simulink model "ex05_target_fio2_track_object_demo"  (Simulink 7.3)
settings: Solver=FixedStepDiscrete  SolverMode=SingleTasking  StartTime=0.0  StopTime=1  RelTol=1e-3
PreLoadFcn:
  | waijung.modelPreload; % Required for working with Waijung Blockset. Do not remove.
undefined symbols (not defined in the file): A1, A2, A7, B10, B11, B12, C1, C2, C3, C4, C5, Custom, G14, H2, H3, H6, H7, Link, LQFP176, ST, STM32F417IG, system_stm32f4xx
libraries: simulink x11, stm32f4_i2c_lib x8, viptextngfix x2, stm32f4_tim_lib x2, waijung_addon_module x2, waijung_webserver x2, dspsigattribs x1, waijung_image_sensor_lib x1, stm32f4_fsmc_lib x1, stm32f4_rcc_lib x1, stm32f4_device_config_lib x1, waijung_socket_lib x1
(part 2 of 2)

== system ex05_target_fio2_track_object_demo/Image Sensor/Camera OV1/Init_/While Iterator_/Picture Size_/Subsystem/Subsystem/Img480x640 ==
  Index : Inport  OutDataType=fixdt(1, 16)  OutScaling=2^0
  Action Port : ActionPort  ActionType=default
  Register List : Subsystem  mask{register=uint8([58,61,140,64,18,50,23,24,25,26,3,12,62,112,113,114,115,162]), value=uint8([8,130,0,208,4,128,22,4,3,123,10,0,0,58,53,17,240,2])}
      mask prompts: register "Register Index"; value "Register Value"
      mask help:
      | Count:
      |  - Number of Register-Value pair.
      |  - Determine from lowest size, between Register and Value.
      | Reg:
      |  - Register index.
      | Value:
      |  - Data corresponding to specified register index.
  Count : Outport  OutDataType=fixdt(1, 16)  OutScaling=2^0
  Reg : Outport  Port=2  OutDataType=fixdt(1, 16)  OutScaling=2^0
  Value : Outport  Port=3  OutDataType=fixdt(1, 16)  OutScaling=2^0
  wires:
  Register List/3(Value) -> Value/1
  Register List/2(Reg) -> Reg/1
  Register List/1(Count) -> Count/1
  Index/1 -> Register List/1(Index)

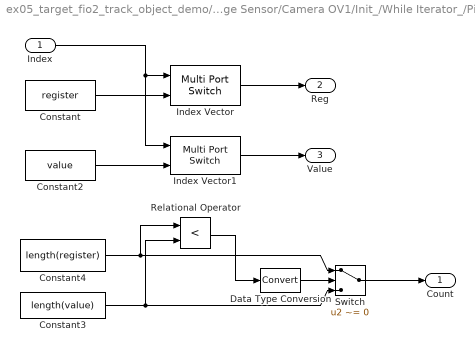
== system ex05_target_fio2_track_object_demo/Image Sensor/Camera OV1/Init_/While Iterator_/Picture Size_/Subsystem/Subsystem/Img120x160/Register List ==
  Index : Inport  OutDataType=fixdt(1, 16)  OutScaling=2^0
  Constant : Constant  Value=register  OutDataType=fixdt(1, 16)  OutScaling=2^0
  Constant2 : Constant  Value=value  OutDataType=fixdt(1, 16)  OutScaling=2^0
  Constant3 : Constant  Value=length(value)  OutDataType=fixdt(1, 16)  OutScaling=2^0
  Constant4 : Constant  Value=length(register)  OutDataType=fixdt(1, 16)  OutScaling=2^0
  Data Type Conversion : DataTypeConversion  OutDataType=fixdt(1, 16)  OutScaling=2^0
  Index Vector : MultiPortSwitch  Inputs=1  zeroidx=on  OutDataType=fixdt(1, 16)  OutScaling=2^0
  Index Vector1 : MultiPortSwitch  Inputs=1  zeroidx=on  OutDataType=fixdt(1, 16)  OutScaling=2^0
  Relational Operator : RelationalOperator  Operator=<  LogicOutDataTypeMode=boolean  LogicDataType=fixdt(0, 8)  OutDataTypeStr=boolean
  Switch : Switch  Criteria=u2 ~= 0  OutDataType=fixdt(1, 16)  OutScaling=2^0
  Count : Outport  OutDataType=fixdt(1, 16)  OutScaling=2^0
  Reg : Outport  Port=2  OutDataType=fixdt(1, 16)  OutScaling=2^0
  Value : Outport  Port=3  OutDataType=fixdt(1, 16)  OutScaling=2^0
  wires:
  Index Vector/1 -> Reg/1
  Constant/1 -> Index Vector/2
  Index/1 -> Index Vector/1, Index Vector1/1
  Constant2/1 -> Index Vector1/2
  Index Vector1/1 -> Value/1
  Constant4/1 -> Relational Operator/1, Switch/1
  Constant3/1 -> Relational Operator/2, Switch/3
  Relational Operator/1 -> Data Type Conversion/1
  Switch/1 -> Count/1
  Data Type Conversion/1 -> Switch/2

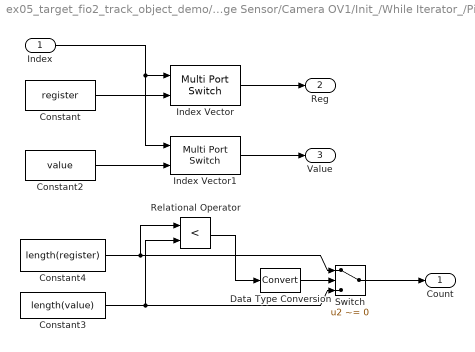
== system ex05_target_fio2_track_object_demo/Image Sensor/Camera OV1/Init_/While Iterator_/Picture Size_/Subsystem/Subsystem/Img240x320/Register List ==
  Index : Inport  OutDataType=fixdt(1, 16)  OutScaling=2^0
  Constant : Constant  Value=register  OutDataType=fixdt(1, 16)  OutScaling=2^0
  Constant2 : Constant  Value=value  OutDataType=fixdt(1, 16)  OutScaling=2^0
  Constant3 : Constant  Value=length(value)  OutDataType=fixdt(1, 16)  OutScaling=2^0
  Constant4 : Constant  Value=length(register)  OutDataType=fixdt(1, 16)  OutScaling=2^0
  Data Type Conversion : DataTypeConversion  OutDataType=fixdt(1, 16)  OutScaling=2^0
  Index Vector : MultiPortSwitch  Inputs=1  zeroidx=on  OutDataType=fixdt(1, 16)  OutScaling=2^0
  Index Vector1 : MultiPortSwitch  Inputs=1  zeroidx=on  OutDataType=fixdt(1, 16)  OutScaling=2^0
  Relational Operator : RelationalOperator  Operator=<  LogicOutDataTypeMode=boolean  LogicDataType=fixdt(0, 8)  OutDataTypeStr=boolean
  Switch : Switch  Criteria=u2 ~= 0  OutDataType=fixdt(1, 16)  OutScaling=2^0
  Count : Outport  OutDataType=fixdt(1, 16)  OutScaling=2^0
  Reg : Outport  Port=2  OutDataType=fixdt(1, 16)  OutScaling=2^0
  Value : Outport  Port=3  OutDataType=fixdt(1, 16)  OutScaling=2^0
  wires:
  Data Type Conversion/1 -> Switch/2
  Switch/1 -> Count/1
  Relational Operator/1 -> Data Type Conversion/1
  Constant3/1 -> Switch/3, Relational Operator/2
  Constant4/1 -> Switch/1, Relational Operator/1
  Index Vector1/1 -> Value/1
  Constant2/1 -> Index Vector1/2
  Index/1 -> Index Vector1/1, Index Vector/1
  Constant/1 -> Index Vector/2
  Index Vector/1 -> Reg/1

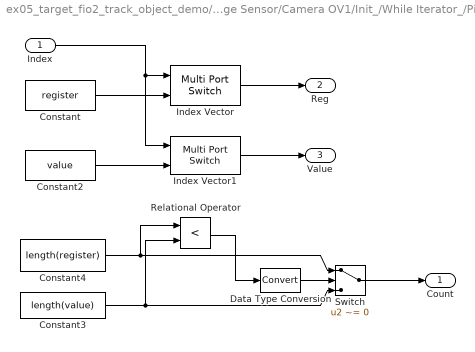
== system ex05_target_fio2_track_object_demo/Image Sensor/Camera OV1/Init_/While Iterator_/Picture Size_/Subsystem/Subsystem/Img480x640/Register List ==
  Index : Inport  OutDataType=fixdt(1, 16)  OutScaling=2^0
  Constant : Constant  Value=register  OutDataType=fixdt(1, 16)  OutScaling=2^0
  Constant2 : Constant  Value=value  OutDataType=fixdt(1, 16)  OutScaling=2^0
  Constant3 : Constant  Value=length(value)  OutDataType=fixdt(1, 16)  OutScaling=2^0
  Constant4 : Constant  Value=length(register)  OutDataType=fixdt(1, 16)  OutScaling=2^0
  Data Type Conversion : DataTypeConversion  OutDataType=fixdt(1, 16)  OutScaling=2^0
  Index Vector : MultiPortSwitch  Inputs=1  zeroidx=on  OutDataType=fixdt(1, 16)  OutScaling=2^0
  Index Vector1 : MultiPortSwitch  Inputs=1  zeroidx=on  OutDataType=fixdt(1, 16)  OutScaling=2^0
  Relational Operator : RelationalOperator  Operator=<  LogicOutDataTypeMode=boolean  LogicDataType=fixdt(0, 8)  OutDataTypeStr=boolean
  Switch : Switch  Criteria=u2 ~= 0  OutDataType=fixdt(1, 16)  OutScaling=2^0
  Count : Outport  OutDataType=fixdt(1, 16)  OutScaling=2^0
  Reg : Outport  Port=2  OutDataType=fixdt(1, 16)  OutScaling=2^0
  Value : Outport  Port=3  OutDataType=fixdt(1, 16)  OutScaling=2^0
  wires:
  Index Vector/1 -> Reg/1
  Constant/1 -> Index Vector/2
  Index/1 -> Index Vector/1, Index Vector1/1
  Constant2/1 -> Index Vector1/2
  Index Vector1/1 -> Value/1
  Constant4/1 -> Relational Operator/1, Switch/1
  Constant3/1 -> Relational Operator/2, Switch/3
  Relational Operator/1 -> Data Type Conversion/1
  Switch/1 -> Count/1
  Data Type Conversion/1 -> Switch/2

== matlab function Embedded MATLAB Function ==
  data: img_in input double; x output double; y output double
function [x,y] = object_tracking(img_in)
	%#eml
	
	persistent ubar
	persistent cnt
	persistent gauss_filt
	
	% Define background image
	if isempty(ubar)
		ubar = single(zeros(size(img_in)));
		cnt = single(0);
		gauss_filt = single([0.0013841   0.0015144   0.0016406   0.0017595   0.0018683   0.0019641   0.0020443   0.0021065   0.0021491   0.0021707   0.0021707   0.0021491   0.0021065   0.0020443   0.0019641   0.0018683   0.0017595   0.0016406   0.0015144   0.0013841
			0.0015144   0.0016571   0.0017951   0.0019252   0.0020443   0.0021491   0.0022368   0.0023049   0.0023515   0.0023751   0.0023751   0.0023515   0.0023049   0.0022368   0.0021491   0.0020443   0.0019252   0.0017951   0.0016571   0.0015144
			0.0016406   0.0017951   0.0019446   0.0020856   0.0022145   0.0023281   0.0024231   0.0024969   0.0025473   0.0025729   0.0025729   0.0025473   0.0024969   0.0024231   0.0023281   0.0022145   0.0020856   0.0019446   0.0017951   0.0016406
			0.0017595   0.0019252   0.0020856   0.0022368   0.0023751   0.0024969   0.0025988   0.0026779    0.002732   0.0027595   0.0027595    0.002732   0.0026779   0.0025988   0.0024969   0.0023751   0.0022368   0.0020856   0.0019252   0.0017595
			0.0018683   0.0020443   0.0022145   0.0023751    0.002522   0.0026513   0.0027595   0.0028435    0.002901   0.0029301   0.0029301    0.002901   0.0028435   0.0027595   0.0026513    0.002522   0.0023751   0.0022145   0.0020443   0.0018683
			0.0019641   0.0021491   0.0023281   0.0024969   0.0026513   0.0027872    0.002901   0.0029893   0.0030497   0.0030804   0.0030804   0.0030497   0.0029893    0.002901   0.0027872   0.0026513   0.0024969   0.0023281   0.0021491   0.0019641
			0.0020443   0.0022368   0.0024231   0.0025988   0.0027595    0.002901   0.0030194   0.0031113   0.0031742   0.0032061   0.0032061   0.0031742   0.0031113   0.0030194    0.002901   0.0027595   0.0025988   0.0024231   0.0022368   0.0020443
			0.0021065   0.0023049   0.0024969   0.0026779   0.0028435   0.0029893   0.0031113   0.0032061   0.0032708   0.0033037   0.0033037   0.0032708   0.0032061   0.0031113   0.0029893   0.0028435   0.0026779   0.0024969   0.0023049   0.0021065
			0.0021491   0.0023515   0.0025473    0.002732    0.002901   0.0030497   0.0031742   0.0032708   0.0033369   0.0033705   0.0033705   0.0033369   0.0032708   0.0031742   0.0030497    0.002901    0.002732   0.0025473   0.0023515   0.0021491
			0.0021707   0.0023751   0.0025729   0.0027595   0.0029301   0.0030804   0.0032061   0.0033037   0.0033705   0.0034043   0.0034043   0.0033705   0.0033037   0.0032061   0.0030804   0.0029301   0.0027595   0.0025729   0.0023751   0.0021707
			0.0021707   0.0023751   0.0025729   0.0027595   0.0029301   0.0030804   0.0032061   0.0033037   0.0033705   0.0034043   0.0034043   0.0033705   0.0033037   0.0032061   0.0030804   0.0029301   0.0027595   0.0025729   0.0023751   0.0021707
			0.0021491   0.0023515   0.0025473    0.002732    0.002901   0.0030497   0.0031742   0.0032708   0.0033369   0.0033705   0.0033705   0.0033369   0.0032708   0.0031742   0.0030497    0.002901    0.002732   0.0025473   0.0023515   0.0021491
			0.0021065   0.0023049   0.0024969   0.0026779   0.0028435   0.0029893   0.0031113   0.0032061   0.0032708   0.0033037   0.0033037   0.0032708   0.0032061   0.0031113   0.0029893   0.0028435   0.0026779   0.0024969   0.0023049   0.0021065
			0.0020443   0.0022368   0.0024231   0.0025988   0.0027595    0.002901   0.0030194   0.0031113   0.0031742   0.0032061   0.0032061   0.0031742   0.0031113   0.0030194    0.002901   0.0027595   0.0025988   0.0024231   0.0022368   0.0020443
			0.0019641   0.0021491   0.0023281   0.0024969   0.0026513   0.0027872    0.002901   0.0029893   0.0030497   0.0030804   0.0030804   0.0030497   0.0029893    0.002901   0.0027872   0.0026513   0.0024969   0.0023281   0.0021491   0.0019641
			0.0018683   0.0020443   0.0022145   0.0023751    0.002522   0.0026513   0.0027595   0.0028435    0.002901   0.0029301   0.0029301    0.002901   0.0028435   0.0027595   0.0026513    0.002522   0.0023751   0.0022145   0.0020443   0.0018683
			0.0017595   0.0019252   0.0020856   0.0022368   0.0023751   0.0024969   0.0025988   0.0026779    0.002732   0.0027595   0.0027595    0.002732   0.0026779   0.0025988   0.0024969   0.0023751   0.0022368   0.0020856   0.0019252   0.0017595
			0.0016406   0.0017951   0.0019446   0.0020856   0.0022145   0.0023281   0.0024231   0.0024969   0.0025473   0.0025729   0.0025729   0.0025473   0.0024969   0.0024231   0.0023281   0.0022145   0.0020856   0.0019446   0.0017951   0.0016406
			0.0015144   0.0016571   0.0017951   0.0019252   0.0020443   0.0021491   0.0022368   0.0023049   0.0023515   0.0023751   0.0023751   0.0023515   0.0023049   0.0022368   0.0021491   0.0020443   0.0019252   0.0017951   0.0016571   0.0015144
			0.0013841   0.0015144   0.0016406   0.0017595   0.0018683   0.0019641   0.0020443   0.0021065   0.0021491   0.0021707   0.0021707   0.0021491   0.0021065   0.0020443   0.0019641   0.0018683   0.0017595   0.0016406   0.0015144   0.0013841]);
	end
	
	cnt = cnt + single(1);
	
	% Subtract background image
	if (cnt <= 20)
		% Find the mean of the back ground image
		ubar = (((cnt-single(1))/cnt)*ubar) + (single(img_in)/cnt);
		img = ubar;
	else
		% Substract background image from current image
		img = single(img_in) - ubar;
	end
	
	% Apply Gaussian Filtering by 2D convolution
	% This algorithm put execessive computation load on the MCU.
	% img = conv2(img,gauss_filt,'same');
	
	% Histogram thresholding
	img_logic = (img < single(-20));
	
	% Find position X Y
	sumx = single(0);
	sumx_cnt = single(0);
	sumy = single(0);
	sumy_cnt = single(0);	
	for j = single(1:2:120) % Skip some pixels to reduce computational load.
		for i = single(1:2:160)
			if (img_logic(i,j) ~= 0)
				sumx = sumx + i;
				sumx_cnt = sumx_cnt + 1;
			end
			if (img_logic(i,j) ~= 0)
				sumy = sumy + j;
				sumy_cnt = sumy_cnt + 1;
			end			
		end
	end
	if (sumx ~= 0)
		x = sumx/sumx_cnt;
	else
		x = single(0);
	end
	
	if (sumy ~= 0)
		y = sumy/sumy_cnt;
	else
		y = single(0);
	end
end
